simulink model "reg_example"  (R2017b)
settings: Solver=VariableStepAuto  StartTime=0.0  StopTime=100e-6  RelTol=1e-3
PreLoadFcn:
  | setup
values from neighbouring files (symbols this model uses):
  axiClk = 156.25e6    (= 156250000)    [setup.m]    (also in setup_exampleModel_bus_axi_simulink.m; setup_exampleModel_bus_axi_simulink_lcls2.m; setup_lcls2_pcav.m; sysgen_signal.m)
  cav1p1_addr = 204    [setup_exampleModel_bus_axi_simulink.m]    (also in setup_exampleModel_bus_axi_simulink_lcls2.m; setup_lcls2_pcav.m; sysgen_signal.m)
  cav1p2_addr = cav1p1_addr * 2    (= 408)    [setup_exampleModel_bus_axi_simulink.m]    (also in setup_exampleModel_bus_axi_simulink_lcls2.m; setup_lcls2_pcav.m; sysgen_signal.m)
  cav2p1_addr = cav1p1_addr * 3    (= 612)    [setup_exampleModel_bus_axi_simulink.m]    (also in setup_exampleModel_bus_axi_simulink_lcls2.m; setup_lcls2_pcav.m; sysgen_signal.m)
  cav2p2_addr = cav1p1_addr * 4    (= 816)    [setup_exampleModel_bus_axi_simulink.m]    (also in setup_exampleModel_bus_axi_simulink_lcls2.m; setup_lcls2_pcav.m; sysgen_signal.m)
  Fadc = Fs/interleavedChannels    (= 29750000)    [setup.m]    (also in setup_exampleModel_bus_axi_simulink.m = 357000000; setup_exampleModel_bus_axi_simulink_lcls2.m = 351000000; setup_lcls2_pcav.m = 357000000; sysgen_signal.m = 357000000)
  Fproc = 204e6    (= 204000000)    [setup_exampleModel_bus_axi_simulink.m]    (also in setup_exampleModel_bus_axi_simulink_lcls2.m = 200571400; setup_lcls2_pcav.m; sysgen_signal.m)
undefined symbols (not defined in the file or in its folder): AXI4, Lite
libraries: xbsIndex_r4 x427, simulink x2
(part 3 of 3)

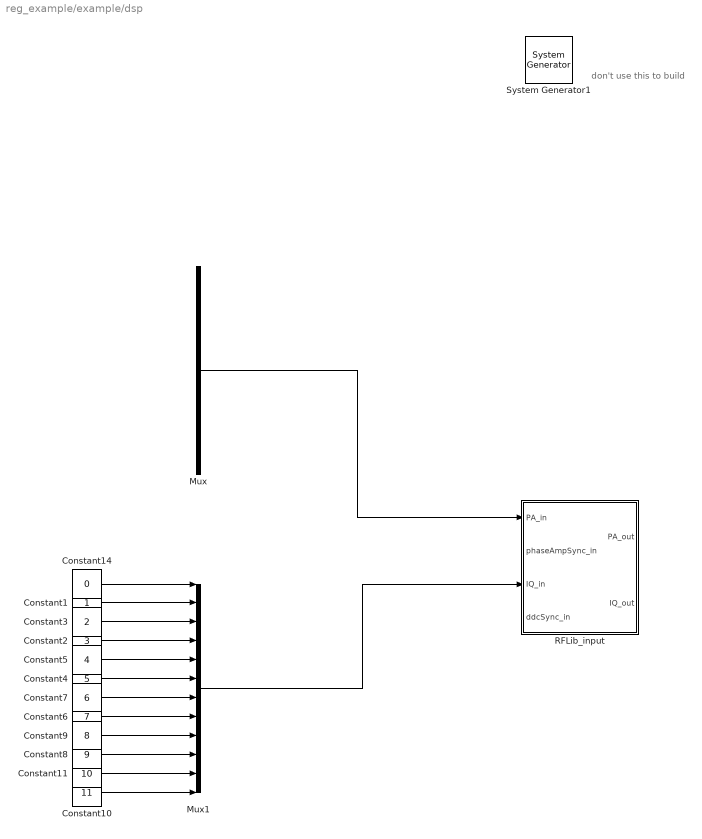
== system reg_example/example/dsp ==
  note: don't use this to build
  " System Generator1" : xbsIndex_r4/ System Generator  Tag=genX  xilinxfamily=kintexu  part=xcku040  speed=-2-e  package=ffva1156  synthesis_tool=Vivado  clock_wrapper=Clock Enables  directory=./netlist  proj_type=Vivado  Synth_file=Vivado Synthesis Defaults  Impl_file=Vivado Implementation Defaults  testbench=off  simulink_period=1/Fproc  sysclk_period=1e9/Fproc  dcm_input_clock_period=10  incr_netlist=off  trim_vbits=Everywhere in SubSystem  dbl_ovrd=According to Block Masks  core_generation=According to Block Masks  run_coregen=off  deprecated_control=off  eval_field=0  block_type=sysgen
  Constant1 : Constant  SampleTime=21/Fadc
  Constant10 : Constant  Value=11  SampleTime=21/Fadc
  Constant11 : Constant  Value=10  SampleTime=21/Fadc
  Constant14 : Constant  Value=0  SampleTime=21/Fadc
  Constant2 : Constant  Value=3  SampleTime=21/Fadc
  Constant3 : Constant  Value=2  SampleTime=21/Fadc
  Constant4 : Constant  Value=5  SampleTime=21/Fadc
  Constant5 : Constant  Value=4  SampleTime=21/Fadc
  Constant6 : Constant  Value=7  SampleTime=21/Fadc
  Constant7 : Constant  Value=6  SampleTime=21/Fadc
  Constant8 : Constant  Value=9  SampleTime=21/Fadc
  Constant9 : Constant  Value=8  SampleTime=21/Fadc
  Mux : Mux  Inputs=12
  Mux1 : Mux  Inputs=12
  RFLib_input : Subsystem
  wires:
  Constant14/1 -> Mux1/1
  Constant1/1 -> Mux1/2
  Constant2/1 -> Mux1/4
  Constant3/1 -> Mux1/3
  Constant7/1 -> Mux1/7
  Constant6/1 -> Mux1/8
  Constant4/1 -> Mux1/6
  Constant5/1 -> Mux1/5
  Constant9/1 -> Mux1/9
  Constant8/1 -> Mux1/10
  Constant10/1 -> Mux1/12
  Constant11/1 -> Mux1/11
  Mux/1 -> RFLib_input/1(PA_in)
  Mux1/1 -> RFLib_input/3(IQ_in)

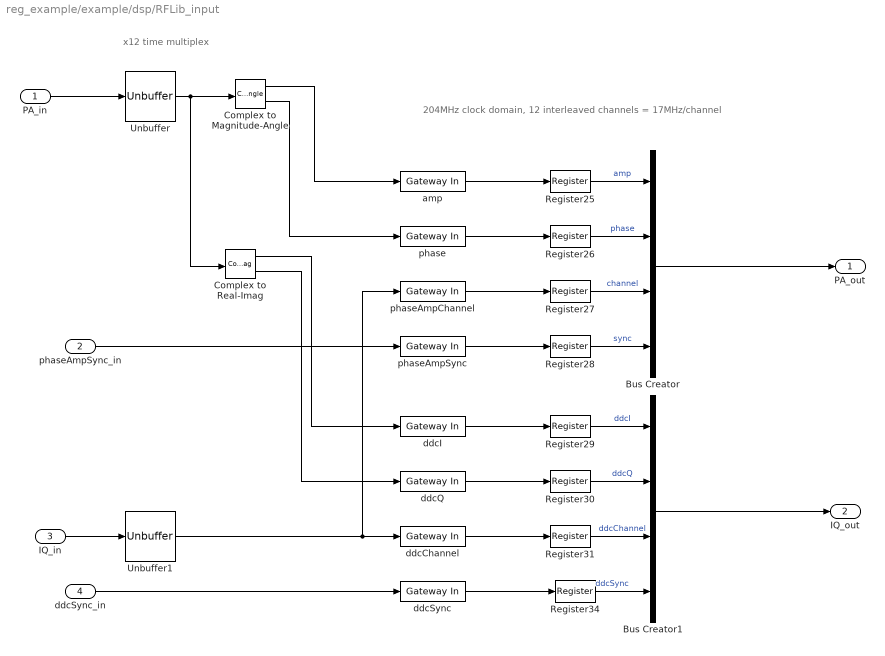
== system reg_example/example/dsp/RFLib_input ==
  note: x12 time multiplex
  note: 204MHz clock domain, 12 interleaved channels = 17MHz/channel
  PA_in : Inport
  phaseAmpSync_in : Inport  Port=2
  IQ_in : Inport  Port=3
  ddcSync_in : Inport  Port=4
  Bus Creator : BusCreator  Inputs=4
  Bus Creator1 : BusCreator  Inputs=4
  Complex to Magnitude-Angle : ComplexToMagnitudeAngle
  Complex to Real-Imag : ComplexToRealImag
  Register{25..31,34} (8 alike) : xbsIndex_r4/Register  init=0  rst=off  en=off  dbl_ovrd=off  block_type=register
  Unbuffer : Unbuffer
  Unbuffer1 : Unbuffer
  amp : xbsIndex_r4/Gateway In  gui_display_data_type=Fixed-point  arith_type="Signed  (2's comp)"  n_bits=18  bin_pt=17  preci_type=Single  exp_width=8  frac_width=24  rows=1  columns=1  quantization="Round  (unbiased: +/- Inf)"  overflow=Saturate  period=1/Fproc  UseAsADC=off  ADCChannel='1'  interface=None  automatic_assignment=on  address_offset=hex2dec('00')  intf_name=''  intf_description=''  default_value=0  timing_constraint=None  locs_specified=off  LOCs={}  io_standard={}  inherit_from_input=off  hdl_port=on  dbl_ovrd=off  block_type=gatewayin
  ddcChannel : xbsIndex_r4/Gateway In  gui_display_data_type=Fixed-point  arith_type=Unsigned  n_bits=4  bin_pt=0  preci_type=Single  exp_width=8  frac_width=24  rows=1  columns=1  quantization="Round  (unbiased: +/- Inf)"  overflow=Saturate  period=1/Fproc  UseAsADC=off  ADCChannel='1'  interface=None  automatic_assignment=on  address_offset=hex2dec('00')  intf_name=''  intf_description=''  default_value=0  timing_constraint=None  locs_specified=off  LOCs={}  io_standard={}  inherit_from_input=off  hdl_port=on  dbl_ovrd=off  block_type=gatewayin
  ddcI : xbsIndex_r4/Gateway In  gui_display_data_type=Fixed-point  arith_type="Signed  (2's comp)"  n_bits=18  bin_pt=17  preci_type=Single  exp_width=8  frac_width=24  rows=1  columns=1  quantization="Round  (unbiased: +/- Inf)"  overflow=Saturate  period=1/Fproc  UseAsADC=off  ADCChannel='1'  interface=None  automatic_assignment=on  address_offset=hex2dec('00')  intf_name=''  intf_description=''  default_value=0  timing_constraint=None  locs_specified=off  LOCs={}  io_standard={}  inherit_from_input=off  hdl_port=on  dbl_ovrd=off  block_type=gatewayin
  ddcQ : xbsIndex_r4/Gateway In  gui_display_data_type=Fixed-point  arith_type="Signed  (2's comp)"  n_bits=18  bin_pt=17  preci_type=Single  exp_width=8  frac_width=24  rows=1  columns=1  quantization="Round  (unbiased: +/- Inf)"  overflow=Saturate  period=1/Fproc  UseAsADC=off  ADCChannel='1'  interface=None  automatic_assignment=on  address_offset=hex2dec('00')  intf_name=''  intf_description=''  default_value=0  timing_constraint=None  locs_specified=off  LOCs={}  io_standard={}  inherit_from_input=off  hdl_port=on  dbl_ovrd=off  block_type=gatewayin
  ddcSync : xbsIndex_r4/Gateway In  gui_display_data_type=Fixed-point  arith_type=Unsigned  n_bits=1  bin_pt=0  preci_type=Single  exp_width=8  frac_width=24  rows=1  columns=1  quantization="Round  (unbiased: +/- Inf)"  overflow=Saturate  period=1/Fproc  UseAsADC=off  ADCChannel='1'  interface=None  automatic_assignment=on  address_offset=hex2dec('00')  intf_name=''  intf_description=''  default_value=0  timing_constraint=None  locs_specified=off  LOCs={}  io_standard={}  inherit_from_input=off  hdl_port=on  dbl_ovrd=off  block_type=gatewayin
  phase : xbsIndex_r4/Gateway In  gui_display_data_type=Fixed-point  arith_type="Signed  (2's comp)"  n_bits=18  bin_pt=17  preci_type=Single  exp_width=8  frac_width=24  rows=1  columns=1  quantization="Round  (unbiased: +/- Inf)"  overflow=Saturate  period=1/Fproc  UseAsADC=off  ADCChannel='1'  interface=None  automatic_assignment=on  address_offset=hex2dec('00')  intf_name=''  intf_description=''  default_value=0  timing_constraint=None  locs_specified=off  LOCs={}  io_standard={}  inherit_from_input=off  hdl_port=on  dbl_ovrd=off  block_type=gatewayin
  phaseAmpChannel : xbsIndex_r4/Gateway In  gui_display_data_type=Fixed-point  arith_type=Unsigned  n_bits=4  bin_pt=0  preci_type=Single  exp_width=8  frac_width=24  rows=1  columns=1  quantization="Round  (unbiased: +/- Inf)"  overflow=Saturate  period=1/Fproc  UseAsADC=off  ADCChannel='1'  interface=None  automatic_assignment=on  address_offset=hex2dec('00')  intf_name=''  intf_description=''  default_value=0  timing_constraint=None  locs_specified=off  LOCs={}  io_standard={}  inherit_from_input=off  hdl_port=on  dbl_ovrd=off  block_type=gatewayin
  phaseAmpSync : xbsIndex_r4/Gateway In  gui_display_data_type=Fixed-point  arith_type=Unsigned  n_bits=1  bin_pt=0  preci_type=Single  exp_width=8  frac_width=24  rows=1  columns=1  quantization="Round  (unbiased: +/- Inf)"  overflow=Saturate  period=1/Fproc  UseAsADC=off  ADCChannel='1'  interface=None  automatic_assignment=on  address_offset=hex2dec('00')  intf_name=''  intf_description=''  default_value=0  timing_constraint=None  locs_specified=off  LOCs={}  io_standard={}  inherit_from_input=off  hdl_port=on  dbl_ovrd=off  block_type=gatewayin
  PA_out : Outport
  IQ_out : Outport  Port=2
  wires:
  phaseAmpSync_in/1 -> phaseAmpSync/1
  amp/1 -> Register25/1
  phase/1 -> Register26/1
  phaseAmpChannel/1 -> Register27/1
  phaseAmpSync/1 -> Register28/1
  ddcI/1 -> Register29/1
  ddcQ/1 -> Register30/1
  ddcChannel/1 -> Register31/1
  PA_in/1 -> Unbuffer/1
  ddcSync/1 -> Register34/1
  Register25/1 -> Bus Creator/1  "amp"
  Register26/1 -> Bus Creator/2  "phase"
  Register27/1 -> Bus Creator/3  "channel"
  Register28/1 -> Bus Creator/4  "sync"
  Register29/1 -> Bus Creator1/1  "ddcI"
  Register30/1 -> Bus Creator1/2  "ddcQ"
  Register31/1 -> Bus Creator1/3  "ddcChannel"
  Register34/1 -> Bus Creator1/4  "ddcSync"
  IQ_in/1 -> Unbuffer1/1
  Unbuffer1/1 -> phaseAmpChannel/1, ddcChannel/1
  Bus Creator/1 -> PA_out/1
  Unbuffer/1 -> Complex to Real-Imag/1, Complex to Magnitude-Angle/1
  Complex to Magnitude-Angle/1 -> amp/1
  Complex to Magnitude-Angle/2 -> phase/1
  Complex to Real-Imag/1 -> ddcI/1
  Complex to Real-Imag/2 -> ddcQ/1
  Bus Creator1/1 -> IQ_out/1
  ddcSync_in/1 -> ddcSync/1
